simulink model "Z_trajectory_plus_else"  (R2018b)
settings: Solver=FixedStepAuto  StartTime=0.0  StopTime=10.0  RelTol=1e-3  EnableMultiTasking=on
undefined symbols (not defined in the file or in its folder): dev, Main, pwm_output0
libraries: simulink x3, px4uORBlib x2, px4Sensorslib x2, px4lib x1
settings Model: SimulationMode=external  ExtModeTrigDuration=10  Creator=Tejas Rajopadhye  LastModifiedBy=Tejas Rajopadhye
settings SolverCC: PositivePriorityOrder=on  AutoInsertRateTranBlk=on
settings OptimizationCC: EnhancedBackFolding=on  PassReuseOutputArgsAs=Individual arguments  MaxStackSize=64  OptimizeBlockOrder=speed  DifferentSizesBufferReuse=on  OptimizationCustomize=off
settings DebuggingCC: ParameterTunabilityLossMsg=error
settings HardwareCC: ProdBitPerPointer=32  ProdBitPerSizeT=32  ProdBitPerPtrDiffT=32  ProdLargestAtomicInteger=Long  ProdLargestAtomicFloat=Double  ProdWordSize=32  ProdLongLongMode=on  ProdHWDeviceType=ARM Compatible->ARM Cortex
settings SFSimCC: MATLABDynamicMemAlloc=off
settings RTWCC: SystemTargetFile=ert.tlc  HardwareBoard=PX4 Pixhawk 4  TLCOptions="-aInlineSetEventsForThisBaseRateFcn=TLC_FALSE -aSuppressMultiTaskScheduler=TLC_FALSE  -aRateBasedStepFcn=0"  TemplateMakefile=ert_default_tmf  GenerateReport=on  Toolchain=GNU Tools for PX4 Autopilots  IncludeHyperlinkInReport=on  LaunchReport=on  TargetLang=C++  GenerateTraceInfo=on  GenerateTraceReport=on  GenerateTraceReportSl=on  GenerateTraceReportSf=on  GenerateTraceReportEml=on
settings CodeAppCC: ForceParamTrailComments=on  IgnoreCustomStorageClasses=off  OperatorAnnotations=on  SimulinkDataObjDesc=on  SFDataObjDesc=on  InsertBlockDesc=on
settings ERTTargetCC: SupportContinuousTime=on

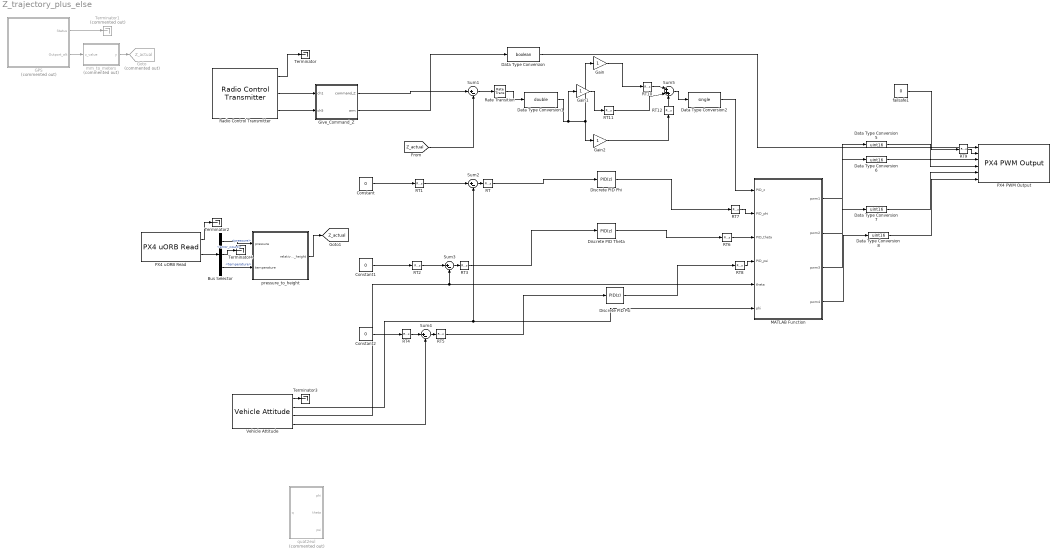
== system Z_trajectory_plus_else ==
  Bus Selector : BusSelector  OutputSignals=pressure,error_count,temperature
  Constant : Constant  Value=0  OutDataTypeStr=uint16  SampleTime=1/250
  Constant1 : Constant  Value=0  OutDataTypeStr=uint16  SampleTime=1/250
  Constant2 : Constant  Value=0  OutDataTypeStr=uint16  SampleTime=1/250
  Data Type Conversion : DataTypeConversion  OutDataTypeStr=boolean
  Data Type Conversion1 : DataTypeConversion  OutDataTypeStr=double
  Data Type Conversion2 : DataTypeConversion  OutDataTypeStr=single
  Data Type Conversion{5..8} (4 alike) : DataTypeConversion  OutDataTypeStr=uint16
  Discrete PID Phi : simulink/Continuous/PID Controller  Controller=PID  Form=Parallel  TimeDomain=Discrete-time  SampleTime=1/250  IntegratorMethod=Forward Euler  FilterMethod=Forward Euler  ControllerParametersSource=internal  P=1  I=1  D=0  UseFilter=on  N=100  TunerSelectOption=Transfer Function Based (PID Tuner App)  InitialConditionSource=internal  InitialConditionForIntegrator=0  InitialConditionForFilter=0  DifferentiatorICPrevScaledInput=0  ExternalReset=none  TrackingMode=off  Kt=1  LimitOutput=off  UpperSaturationLimit=inf  LowerSaturationLimit=-inf  LinearizeAsGain=off  AntiWindupMode=none  Kb=1  POutMin=[]  POutMax=[]  IOutMin=[]  IOutMax=[]  DOutMin=[]  DOutMax=[]  NOutMin=[]  NOutMax=[]  SumOutMin=[]  SumOutMax=[]  SaturationOutMin=[]  SaturationOutMax=[]  PParamMin=[]  PParamMax=[]  IParamMin=[]  IParamMax=[]  DParamMin=[]  DParamMax=[]  NParamMin=[]  NParamMax=[]  KbParamMin=[]  KbParamMax=[]  KtParamMin=[]  KtParamMax=[]  KbOutMin=[]  KbOutMax=[]  KtOutMin=[]  KtOutMax=[]  IntegratorOutMin=[]  IntegratorOutMax=[]  FilterOutMin=[]  FilterOutMax=[]  SumI1OutMin=[]  SumI1OutMax=[]  SumI2OutMin=[]  SumI2OutMax=[]  SumI3OutMin=[]  SumI3OutMax=[]  SumI4OutMin=[]  SumI4OutMax=[]  SumDOutMin=[]  SumDOutMax=[]  DifferentiatorOutMin=[]  DifferentiatorOutMax=[]  FilterDiffOutCoefMin=[]  FilterDiffOutCoefMax=[]  ReciprocalOutMin=[]  ReciprocalOutMax=[]  SumDenOutMin=[]  SumDenOutMax=[]  SumNumOutMin=[]  SumNumOutMax=[]  DivideOutMin=[]  DivideOutMax=[]  IntegratorContinuousStateAttributes=''  IntegratorStateMustResolveToSignalObject=off  IntegratorRTWStateStorageClass=Auto  FilterContinuousStateAttributes=''  FilterStateMustResolveToSignalObject=off  FilterRTWStateStorageClass=Auto  ParallelPVariant=InternalParameters  IdealPVariant=Disabled  IVariant=InternalParameters  DVariant=InternalParameters  IntegratorVariant=Discrete  SatVariant=Disabled  AWVariant=Passthrough  PCopyVariant=Disabled  TRVariant=Disabled  FdbkBlocksVariant=Forward  IdealPFdbkVariant=Disabled  SatFdbkVariant=Disabled  DerivativeFilterVariant=ForwardEulerFilter  NVariant=InternalParameters  NCopyVariant=Disabled  FilterICVariant=InternalICsFilter  IntegratorICVariant=InternalICs  ExternalResetVariant=Disabled  TRSumVariant=Passthrough  SumFdbkVariant=Disabled  SumVariant=Sum_PID
  Discrete PID Psi : simulink/Continuous/PID Controller  Controller=PID  Form=Parallel  TimeDomain=Discrete-time  SampleTime=1/250  IntegratorMethod=Forward Euler  FilterMethod=Forward Euler  ControllerParametersSource=internal  P=1  I=1  D=0  UseFilter=on  N=100  TunerSelectOption=Transfer Function Based (PID Tuner App)  InitialConditionSource=internal  InitialConditionForIntegrator=0  InitialConditionForFilter=0  DifferentiatorICPrevScaledInput=0  ExternalReset=none  TrackingMode=off  Kt=1  LimitOutput=off  UpperSaturationLimit=inf  LowerSaturationLimit=-inf  LinearizeAsGain=off  AntiWindupMode=none  Kb=1  POutMin=[]  POutMax=[]  IOutMin=[]  IOutMax=[]  DOutMin=[]  DOutMax=[]  NOutMin=[]  NOutMax=[]  SumOutMin=[]  SumOutMax=[]  SaturationOutMin=[]  SaturationOutMax=[]  PParamMin=[]  PParamMax=[]  IParamMin=[]  IParamMax=[]  DParamMin=[]  DParamMax=[]  NParamMin=[]  NParamMax=[]  KbParamMin=[]  KbParamMax=[]  KtParamMin=[]  KtParamMax=[]  KbOutMin=[]  KbOutMax=[]  KtOutMin=[]  KtOutMax=[]  IntegratorOutMin=[]  IntegratorOutMax=[]  FilterOutMin=[]  FilterOutMax=[]  SumI1OutMin=[]  SumI1OutMax=[]  SumI2OutMin=[]  SumI2OutMax=[]  SumI3OutMin=[]  SumI3OutMax=[]  SumI4OutMin=[]  SumI4OutMax=[]  SumDOutMin=[]  SumDOutMax=[]  DifferentiatorOutMin=[]  DifferentiatorOutMax=[]  FilterDiffOutCoefMin=[]  FilterDiffOutCoefMax=[]  ReciprocalOutMin=[]  ReciprocalOutMax=[]  SumDenOutMin=[]  SumDenOutMax=[]  SumNumOutMin=[]  SumNumOutMax=[]  DivideOutMin=[]  DivideOutMax=[]  IntegratorContinuousStateAttributes=''  IntegratorStateMustResolveToSignalObject=off  IntegratorRTWStateStorageClass=Auto  FilterContinuousStateAttributes=''  FilterStateMustResolveToSignalObject=off  FilterRTWStateStorageClass=Auto  ParallelPVariant=InternalParameters  IdealPVariant=Disabled  IVariant=InternalParameters  DVariant=InternalParameters  IntegratorVariant=Discrete  SatVariant=Disabled  AWVariant=Passthrough  PCopyVariant=Disabled  TRVariant=Disabled  FdbkBlocksVariant=Forward  IdealPFdbkVariant=Disabled  SatFdbkVariant=Disabled  DerivativeFilterVariant=ForwardEulerFilter  NVariant=InternalParameters  NCopyVariant=Disabled  FilterICVariant=InternalICsFilter  IntegratorICVariant=InternalICs  ExternalResetVariant=Disabled  TRSumVariant=Passthrough  SumFdbkVariant=Disabled  SumVariant=Sum_PID
  Discrete PID Theta : simulink/Continuous/PID Controller  Controller=PID  Form=Parallel  TimeDomain=Discrete-time  SampleTime=1/250  IntegratorMethod=Forward Euler  FilterMethod=Forward Euler  ControllerParametersSource=internal  P=1  I=1  D=0  UseFilter=on  N=100  TunerSelectOption=Transfer Function Based (PID Tuner App)  InitialConditionSource=internal  InitialConditionForIntegrator=0  InitialConditionForFilter=0  DifferentiatorICPrevScaledInput=0  ExternalReset=none  TrackingMode=off  Kt=1  LimitOutput=off  UpperSaturationLimit=inf  LowerSaturationLimit=-inf  LinearizeAsGain=off  AntiWindupMode=none  Kb=1  POutMin=[]  POutMax=[]  IOutMin=[]  IOutMax=[]  DOutMin=[]  DOutMax=[]  NOutMin=[]  NOutMax=[]  SumOutMin=[]  SumOutMax=[]  SaturationOutMin=[]  SaturationOutMax=[]  PParamMin=[]  PParamMax=[]  IParamMin=[]  IParamMax=[]  DParamMin=[]  DParamMax=[]  NParamMin=[]  NParamMax=[]  KbParamMin=[]  KbParamMax=[]  KtParamMin=[]  KtParamMax=[]  KbOutMin=[]  KbOutMax=[]  KtOutMin=[]  KtOutMax=[]  IntegratorOutMin=[]  IntegratorOutMax=[]  FilterOutMin=[]  FilterOutMax=[]  SumI1OutMin=[]  SumI1OutMax=[]  SumI2OutMin=[]  SumI2OutMax=[]  SumI3OutMin=[]  SumI3OutMax=[]  SumI4OutMin=[]  SumI4OutMax=[]  SumDOutMin=[]  SumDOutMax=[]  DifferentiatorOutMin=[]  DifferentiatorOutMax=[]  FilterDiffOutCoefMin=[]  FilterDiffOutCoefMax=[]  ReciprocalOutMin=[]  ReciprocalOutMax=[]  SumDenOutMin=[]  SumDenOutMax=[]  SumNumOutMin=[]  SumNumOutMax=[]  DivideOutMin=[]  DivideOutMax=[]  IntegratorContinuousStateAttributes=''  IntegratorStateMustResolveToSignalObject=off  IntegratorRTWStateStorageClass=Auto  FilterContinuousStateAttributes=''  FilterStateMustResolveToSignalObject=off  FilterRTWStateStorageClass=Auto  ParallelPVariant=InternalParameters  IdealPVariant=Disabled  IVariant=InternalParameters  DVariant=InternalParameters  IntegratorVariant=Discrete  SatVariant=Disabled  AWVariant=Passthrough  PCopyVariant=Disabled  TRVariant=Disabled  FdbkBlocksVariant=Forward  IdealPFdbkVariant=Disabled  SatFdbkVariant=Disabled  DerivativeFilterVariant=ForwardEulerFilter  NVariant=InternalParameters  NCopyVariant=Disabled  FilterICVariant=InternalICsFilter  IntegratorICVariant=InternalICs  ExternalResetVariant=Disabled  TRSumVariant=Passthrough  SumFdbkVariant=Disabled  SumVariant=Sum_PID
  GPS : Subsystem  Commented=on  mask(Vehicle GPS){lat=off, lon=off, alt=on, velocity=off, gpsfix=off, numsat=off, timestamp=off, BlockingMode=off, BlockTimeout=1e-3, sampleTime=1/250}
      mask prompts: lat "Latitude (1e-7 degress)"; lon "Longitude (1e-7 degress)"; alt "Altitude (mm)"; velocity "Velocity (m/s)"; gpsfix "GPS Fix Type"; numsat "Number of satellites"; timestamp "Timestamp (microseconds)"; BlockingMode "px4:blockmask:SubscriberBlockingMode"; BlockTimeout "px4:blockmask:SubscriberBlockingModeTimeout"; sampleTime "px4:blockmask:SampleTimePrompt"
      mask help:
      | Read Vehicle GPS values using 'vehicle_gps_position' uORB topic.  Select the required GPS values from the list below.
      |
      | Status is a boolean value indicating whether a GPS values was received during the previous time step. When Status is 0, GPS values holds the newly-received message. When Status is 1, GPS values holds the last received message.
      | The Latitude, Longitude and Altitude are scalar values of datatype int32 and Velocity is of datatype single. GPS Fix Type and Number of satellites are scalars of datatype uint8.
      | The Timestamp is the absolute time value when the last message was recieved and is a scalar of datatype uint64.
      mask init:
      | % List of signals required as output
      | signal_names = {'<lat>','<lon>','<alt>','<vel_m_s>','<fix_type>',...
      |                         '<satellites_used>','<timestamp>'};
      | %Output port names to display in the mask
      | output_port_names = {'Latitude','Longitude','Altitude',...
      |                         'Velocity','Fix Type','Num Satellites',...
      |                         'Timestamp'};
      | %Fullpath to the mask image
      | mask_image = [];
      | px4.internal.block.CommonuORBTopicMask.commonMaskCallback(gcb,signal_names,output_port_names,mask_image);
      mask Help: eval('codertarget.internal.helpView(''px4'',''px4vehiclegps'')');
      mask TypeOptions BlockingMode: PX4 uORB Read/BlockingMode
      mask Callback BlockingMode: px4.internal.block.CommonuORBTopicMask.blockingModeCallback(gcb);
      mask TypeOptions BlockTimeout: PX4 uORB Read/BlockTimeout
      mask TypeOptions sampleTime: PX4 uORB Read/sampleTime
      mask DialogControl Container6 Prompt: Main
      mask DialogControl Container11 Prompt: Advanced
      mask DialogControl BlockingMode Prompt: Wait until data received
      mask DialogControl BlockTimeout Prompt: Timeout in seconds:
      mask DialogControl sampleTime Prompt: Sample time (-1 for inherited):
      mask Display:
      | color('blue');
      | text(0.25, 0.9, 'PX4', 'horizontalAlignment', 'right');
      | color('black');
      | text(0.5, 0.5, get_param(gcb,'MaskType'), 'horizontalAlignment', 'center');
      | port_label('output',1,'Status');
      | port_label('output',2,'Altitude');
  Gain : Gain
  Gain1 : Gain
  Gain2 : Gain
  Give_Command_Z : MATLAB Function  TreatAsAtomicUnit=on
  Goto : Goto  Commented=on  GotoTag=Z_actual  TagVisibility=global
  MATLAB Function : MATLAB Function  TreatAsAtomicUnit=on
  PX4 PWM Output : px4lib/PX4 PWM Output  pwmDevice=Main (/dev/pwm_output0)  pwmChannel1_=on  pwmChannel2_=on  pwmChannel3_=on  pwmChannel4_=on  pwmChannel5_=off  pwmChannel6_=off  pwmChannel7_=off  pwmChannel8_=off  forceTerminateFailsafe=off  outputErrorStatus=off
      settings: SourceProductName=Embedded Coder Support Package for PX4 Autopilots  SourceProductBaseCode=PX4AUTOPILOTS
  PX4 uORB Read : px4uORBlib/PX4 uORB Read  uORBTopic=sensor_baro  sampleTime=-1  BlockingMode=off  BlockTimeout=1e-3
      settings: SourceProductName=Embedded Coder Support Package for PX4 Autopilots
  RT : RateTransition  OutPortSampleTime=0.004
  RT{1..2,4,6..12} (10 alike) : RateTransition  OutPortSampleTime=0.002
  RT3 : RateTransition  OutPortSampleTime=0.004
  RT5 : RateTransition  OutPortSampleTime=0.004
  Radio Control Transmitter : px4Sensorslib/Radio Control Transmitter  channel1=on  channel2=off  channel3=off  channel4=off  channel5=on  channel6=off  channel7=off  channel8=off  channel_count=off  rssi=off  rc_input_source=off  timestamp_last_signal=off  time_stamp=off  sampleTime=-1  BlockingMode=off  BlockTimeout=5
      settings: SourceProductName=Embedded Coder Support Package for PX4 Autopilots
  Rate Transition : RateTransition  OutPortSampleTime=0.004
  Sum{1..4} (4 alike) : Sum  Inputs=|+-
  Sum5 : Sum  Inputs=|+++
  Terminator{,2..4} (4 alike) : Terminator
  Terminator1 : Terminator  Commented=on
  Vehicle Attitude : px4Sensorslib/Vehicle Attitude  rollRate=on  pitchRate=on  yawRate=on  quaternion=off  uorbTimeStamp=off  BlockingMode=off  BlockTimeout=0.001  sampleTime=-1
      settings: SourceProductName=Embedded Coder Support Package for PX4 Autopilots
  failsafe1 : Constant  Value=0  OutDataTypeStr=boolean  SampleTime=0.01
  mm_to_meters : MATLAB Function  Commented=on  TreatAsAtomicUnit=on
  pressure_to_height : MATLAB Function  TreatAsAtomicUnit=on
  quat2eul : MATLAB Function  Commented=on  TreatAsAtomicUnit=on
  tag scope: Z_actual=global
  wires:
  Radio Control Transmitter/1 -> Terminator/1
  Radio Control Transmitter/2 -> Give_Command_Z/1(ch1)
  Give_Command_Z/1(command_Z) -> Sum1/1
  GPS/1(Status) -> Terminator1/1
  Data Type Conversion2/1 -> MATLAB Function/1(PID_z)
  MATLAB Function/1(pwm1) -> Data Type Conversion5/1
  MATLAB Function/2(pwm2) -> Data Type Conversion6/1
  MATLAB Function/3(pwm3) -> Data Type Conversion7/1
  MATLAB Function/4(pwm4) -> Data Type Conversion8/1
  Radio Control Transmitter/3 -> Give_Command_Z/2(ch5)
  Give_Command_Z/2(arm) -> Data Type Conversion/1
  failsafe1/1 -> RT9/1
  Data Type Conversion5/1 -> PX4 PWM Output/3
  Data Type Conversion8/1 -> PX4 PWM Output/6
  Data Type Conversion6/1 -> PX4 PWM Output/4
  Data Type Conversion/1 -> PX4 PWM Output/1
  Data Type Conversion7/1 -> PX4 PWM Output/5
  Vehicle Attitude/1 -> Terminator3/1
  [Z_actual] -> Sum1/2
  Constant/1 -> RT1/1
  RT/1 -> Discrete PID Phi/1
  Constant1/1 -> RT2/1
  RT3/1 -> Discrete PID Theta/1
  Constant2/1 -> RT4/1
  RT5/1 -> Discrete PID Psi/1
  Discrete PID Phi/1 -> RT7/1
  Discrete PID Theta/1 -> RT6/1
  Discrete PID Psi/1 -> RT8/1
  GPS/2(Outport_alt) -> mm_to_meters/1(z_value)
  mm_to_meters/1(y) -> Goto/1
  Vehicle Attitude/2 -> MATLAB Function/6(phi), Sum2/2
  Vehicle Attitude/3 -> MATLAB Function/5(theta), Sum3/2
  Vehicle Attitude/4 -> Sum4/2
  Data Type Conversion1/1 -> Gain2/1, Gain/1, Gain1/1
  Sum5/1 -> Data Type Conversion2/1
  PX4 uORB Read/2 -> Bus Selector/1
  Bus Selector/3 -> pressure_to_height/2(temperature)  "<temperature>"
  Bus Selector/2 -> Terminator4/1  "<error_count>"
  PX4 uORB Read/1 -> Terminator2/1
  RT1/1 -> Sum2/1
  RT2/1 -> Sum3/1
  RT4/1 -> Sum4/1
  RT6/1 -> MATLAB Function/3(PID_theta)
  RT7/1 -> MATLAB Function/2(PID_phi)
  RT8/1 -> MATLAB Function/4(PID_psi)
  RT9/1 -> PX4 PWM Output/2
  pressure_to_height/1(relative_height) -> [Z_actual]
  Bus Selector/1 -> pressure_to_height/1(pressure)  "<pressure>"
  Sum1/1 -> Rate Transition/1
  Rate Transition/1 -> Data Type Conversion1/1
  Gain2/1 -> RT12/1
  Sum2/1 -> RT/1
  Sum3/1 -> RT3/1
  Sum4/1 -> RT5/1
  Gain/1 -> RT10/1
  RT11/1 -> Sum5/2
  Gain1/1 -> RT11/1
  RT10/1 -> Sum5/1
  RT12/1 -> Sum5/3

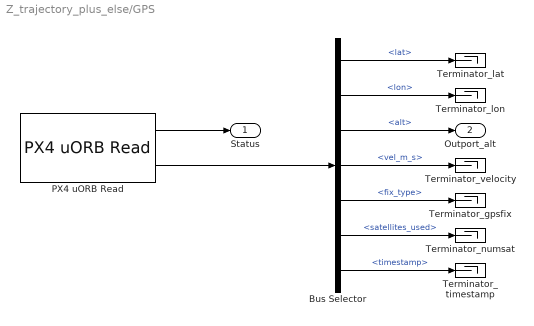
== system Z_trajectory_plus_else/GPS ==
  Bus Selector : BusSelector  OutputSignals=lat,lon,alt,vel_m_s,fix_type,satellites_used,timestamp
  PX4 uORB Read : px4uORBlib/PX4 uORB Read  uORBTopic=vehicle_gps_position  sampleTime=sampleTime  BlockingMode=off  BlockTimeout=BlockTimeout
      settings: SourceProductName=Embedded Coder Support Package for PX4 Autopilots
  Terminator_gpsfix : Terminator
  Terminator_lat : Terminator
  Terminator_lon : Terminator
  Terminator_numsat : Terminator
  Terminator_timestamp : Terminator
  Terminator_velocity : Terminator
  Status : Outport
  Outport_alt : Outport  Port=2
  wires:
  Bus Selector/2 -> Terminator_lon/1  "<lon>"
  Bus Selector/1 -> Terminator_lat/1  "<lat>"
  Bus Selector/7 -> Terminator_timestamp/1  "<timestamp>"
  Bus Selector/6 -> Terminator_numsat/1  "<satellites_used>"
  Bus Selector/5 -> Terminator_gpsfix/1  "<fix_type>"
  Bus Selector/4 -> Terminator_velocity/1  "<vel_m_s>"
  Bus Selector/3 -> Outport_alt/1  "<alt>"
  PX4 uORB Read/1 -> Status/1
  PX4 uORB Read/2 -> Bus Selector/1

== matlab function Z_trajectory_plus_else/MATLAB Function ==
  data: PID_z input; PID_phi input; PID_theta input; PID_psi input; pwm1 output; pwm2 output; pwm3 output; pwm4 output; theta input; phi input
function [pwm1, pwm2, pwm3, pwm4] = pwm_out(PID_z, PID_phi, PID_theta, PID_psi ,theta, phi)
Ixx = single(0.047);
Iyy = single(0.047);
Izz = single(0.094);

g = single(9.81);
l = single(0.225);

ct = single(0.0984);    % Values from doc
cm = single(0.00679);   % Values from doc

%Complete the instrutions
T = g + PID_z /(cos(theta)*cos(phi)); %U4 This is a more logical way of writing the torque term
tauphi = PID_phi*Ixx;
tautheta = PID_theta*Iyy;
taupsi = PID_psi*Izz;

% w1 w2 .... Made changes in the signs according to our calculations and
% model... make sure you do the right connections on the setup

w1 = T/(4*ct) - tautheta/(2*ct*l) - taupsi/(4*cm);
w2 = T/(4*ct) - tauphi/(2*ct*l) + taupsi/(4*cm);
w3 = T/(4*ct) + tautheta/(2*ct*l) - taupsi/(4*cm);
w4 = T/(4*ct) + tauphi/(2*ct*l) + taupsi/(4*cm);


% Taking sqrt of all omega's
w1 = sqrt(w1);
w2 = sqrt(w2);
w3 = sqrt(w3);
w4 = sqrt(w4);


% convert omegas to Pwm values and give the output to pwm block
% From this answer that i got from net about working of ESC's (https://electronics.stackexchange.com/questions/42616/how-to-use-an-esc)
% 100 % Pwm --> 2.0ms (@50hz) --> maxSpeed (11000rpm)
% Using that logic 2,5ms*Xrpm/ 11000rpm will give us the required PWM

pwm1 = (w1*2.0e-3)/11000;
pwm2 = (w2*2.0e-3)/11000;
pwm3 = (w3*2.0e-3)/11000;
pwm4 = (w4*2.0e-3)/11000;

if (pwm1 < single(900) || pwm2 < single(900) || pwm3 < single(900) || pwm4 < single(900))
    pwm1 = single(900);
    pwm2 = single(900);
    pwm3 = single(900);
    pwm4 = single(900);
end
[pwm1, pwm2, pwm3, pwm4];

== matlab function Z_trajectory_plus_else/Give_Command_Z ==
  data: ch1 input; command_Z output; ch5 input; arm output
function [command_Z, arm] = Commands(ch1, ch5)
ch1 = single(ch1);
command_Z = (ch1 - 1000)/100; %for z trajecctory from 0 to 10m
if (ch5 > uint16(1000))
    arm = true;
else
    arm = false;
end
[command_Z, arm];

== matlab function Z_trajectory_plus_else/mm_to_meters ==
  data: z_value input; y output
function y = mm_to_m(z_value)
z_value = single(z_value/10);
y = z_value;

== matlab function Z_trajectory_plus_else/pressure_to_height ==
  data: pressure input; relative_height output; temperature input
function relative_height = covert_pressure_to_height(pressure, temperature)
R = 287;
g = 9.81;
persistent itr;
if isempty(itr)
    itr = 0;
end
persistent init_pressure;
if isempty(init_pressure)
    init_pressure = single(0);
end

if (itr == 0)
    initial_pressure = pressure;
    itr = itr + 1;
else
    initial_pressure = single(init_pressure);
end
if (isreal(log(pressure/initial_pressure)))
    log_value = log(pressure/initial_pressure);
else
    log_value = 0;
end
init_pressure = single(initial_pressure);

relative_height = single(((R*temperature)/g)*log_value);

== matlab function Z_trajectory_plus_else/quat2eul ==
  data: q input; phi output; theta output; psi output
function [phi,theta,psi] = quat2eul(q)
% Conversion from Quaternion to Euler angles based on the PX4 Firmware
% v1.6.5 release.
% 
% Quaternion -> DCM -> Euler Angles
% INPUT:
%   q: Quaternion vector of the format: (a + bi + cj + dk)
% OUTPUT:
%   [phi,theta,psi]: Euler angles in radians.
% 
 
    a = q(1);
    b = q(2);
    c = q(3);
    d = q(4);

    aSq = a*a;
    bSq = b*b;
    cSq = c*c;
    dSq = d*d;

    d_pi2 = pi/2;

    % quaternion_to_dcm
    dcm00 = aSq + bSq - cSq - dSq;
    % dcm01 = 2*(b*c - a*d);
    dcm02 = 2*(a*c + b*d);
    dcm10 = 2*(b*c + a*d);
    % dcm11 = aSq - bSq + cSq - dSq;
    dcm12 = 2*(c*d - a*b);
    dcm20 = 2*(b*d - a*c);
    dcm21 = 2*(a*b + c*d);
    dcm22 = aSq - bSq - cSq + dSq;

    % dcm_to_euler
    theta = asin(-dcm20);
    if abs(theta - d_pi2) < 1.0e-3
        phi = single(0.0);
        psi = atan2(dcm12, dcm02);
    elseif abs(theta + d_pi2) < 1.0e-3
        phi = single(0.0);
        psi = atan2(-dcm12, -dcm02);
    else
        phi = atan2(dcm21, dcm22);
        psi = atan2(dcm10, dcm00);
    end

end
